simulink model "test_PID_function"  (R2015a)
settings: Solver=ode45  StartTime=0.02  StopTime=100.0  FixedStep=0  RelTol=1e-3
libraries: discretizing x2, simulink x1
settings Model: Creator=Dorota  LastModifiedBy=Dorota
settings SFSimCC: SimCustomInitializer=init_test();  SimBuildMode=sf_make_clean
settings SFSimCC: SimCustomHeaderCode=|
  | #include "./PID.h"
  | #include "./test.h"
settings SFSimCC: SimUserSources=|
  | ./PID.c
  | ./test.c

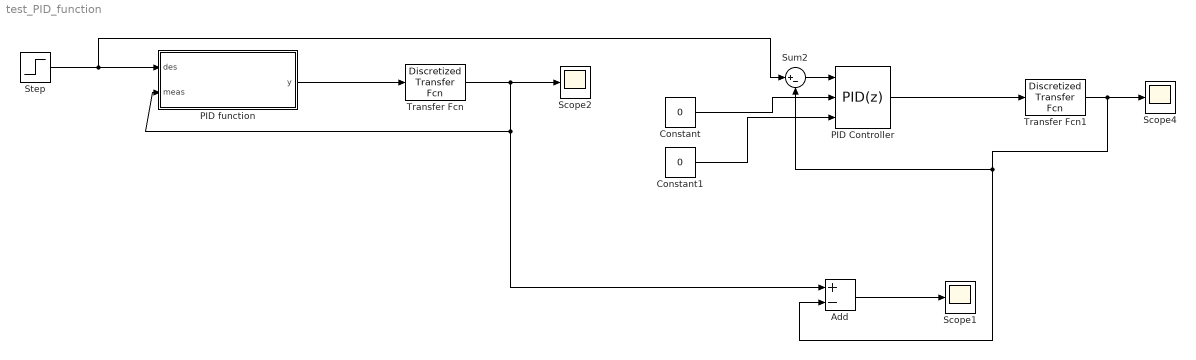
== system test_PID_function ==
  Add : Sum  Inputs=+-
  Constant : Constant  Value=0
  Constant1 : Constant  Value=0
  PID Controller : simulink/Continuous/PID Controller  Controller=PID  TimeDomain=Discrete-time  SampleTime=0.020000000000000001  IntegratorMethod=Forward Euler  FilterMethod=Forward Euler  Form=Parallel  UseFilter=on  ControllerParametersSource=internal  P=0.000478  I=0.0478  D=0  N=100  InitialConditionSource=external  InitialConditionForIntegrator=0  InitialConditionForFilter=0  ExternalReset=none  LimitOutput=off  UpperSaturationLimit=inf  LowerSaturationLimit=-inf  LinearizeAsGain=on  AntiWindupMode=none  Kb=1  TrackingMode=off  Kt=1  PParamMin=[]  PParamMax=[]  IParamMin=[]  IParamMax=[]  DParamMin=[]  DParamMax=[]  NParamMin=[]  NParamMax=[]  KbParamMin=[]  KbParamMax=[]  KtParamMin=[]  KtParamMax=[]  POutMin=[]  POutMax=[]  IOutMin=[]  IOutMax=[]  DOutMin=[]  DOutMax=[]  NOutMin=[]  NOutMax=[]  KbOutMin=[]  KbOutMax=[]  KtOutMin=[]  KtOutMax=[]  IntegratorOutMin=[]  IntegratorOutMax=[]  FilterOutMin=[]  FilterOutMax=[]  SumOutMin=[]  SumOutMax=[]  SumI1OutMin=[]  SumI1OutMax=[]  SumI2OutMin=[]  SumI2OutMax=[]  SumI3OutMin=[]  SumI3OutMax=[]  SumDOutMin=[]  SumDOutMax=[]  SaturationOutMin=[]  SaturationOutMax=[]  IntegratorContinuousStateAttributes=''  IntegratorStateMustResolveToSignalObject=off  IntegratorRTWStateStorageClass=Auto  FilterContinuousStateAttributes=''  FilterStateMustResolveToSignalObject=off  FilterRTWStateStorageClass=Auto  DifferentiatorICPrevScaledInput=0  DifferentiatorOutMin=[]  DifferentiatorOutMax=[]
  PID function : MATLAB Function  TreatAsAtomicUnit=on
  Scope1 : Scope
  Scope2 : Scope
      settings: SaveName=ScopeData2
  Scope4 : Scope
      settings: SaveName=ScopeData4
  Step : Step  SampleTime=0.02  mask(DiscretizedSource){}
      mask init:
      | %zoh
  Sum2 : Sum  Inputs=|+-
  Transfer Fcn : discretizing/Discretized Transfer Fcn  Numerator=[1]  Denominator=[1 0.1 1]  AbsTol=auto  SampleTime=0.02  method=zoh  Wc=1
  Transfer Fcn1 : discretizing/Discretized Transfer Fcn  Numerator=[1]  Denominator=[1 0.1 1]  AbsTol=auto  SampleTime=0.02  method=zoh  Wc=1
  wires:
  PID function/1(y) -> Transfer Fcn/1
  Transfer Fcn/1 -> PID function/2(meas), Add/1, Scope2/1
  Transfer Fcn1/1 -> Add/2, Sum2/2, Scope4/1
  Step/1 -> Sum2/1, PID function/1(des)
  PID Controller/1 -> Transfer Fcn1/1
  Sum2/1 -> PID Controller/1
  Add/1 -> Scope1/1
  Constant/1 -> PID Controller/2
  Constant1/1 -> PID Controller/3

== matlab function test_PID_function/PID function ==
  data: y output; des input; meas input

function y = test (des, meas)
    y = double(0);
    y = coder.ceval('test', 0, single(des), single(meas));
end
